simulink model "AGC30_PVcut_2021"  (R2021a)
settings: Solver=ode4  StartTime=stime  StopTime=etime  FixedStep=dtload  RelTol=1e-3
values from neighbouring files (symbols this model uses):
  AL_A = 0.3    [initset_lfc.m]
  AL_B = 0.3    [initset_lfc.m]
  DELTA_B = 0.067    [initset_otherarea.m]
  dtload = 0.1    [initset_dataload.m]
  F0 = 60    [initset_inertia.m]
  FFCS0_CC = (WF0_CC-WF_MIN_CC)./(1.0-WF_MIN_CC)    [init_thermals.m]
  FX_FB_ST_OA = Fx_fb_st_ty(:,TY_ST)    [initset_otherarea.m]
  FX_FB_WT = FX_FB_WT_ty(:,TY_WT)    [read_const_conhydros.m]
  FX_PTHD_ST_OA = Fx_pthd_st_ty(:,TY_ST)    [initset_otherarea.m]
  FY_FB_ST_OA = [1;1;0;0;-1;-1]*PLM_B    [initset_otherarea.m]
  FY_FB_WT = FY_FB_WT_ty(:,TY_WT)    [read_const_conhydros.m]
  FY_PTHD_ST_OA = [1;1;1;1]    [initset_otherarea.m]
  G_cost = [Cost(:,3) ... (first row only)    [initset_dataload.m]
  G_down_limit = max(G_down_limit, G_out_pre - G_speed*5)    [edc.m]    (also in initset_dataload.m = csvread('G_down_plan_limit.csv',0,1))
  G_G_ST_OA = G_g_st_ty(TY_ST)    [initset_otherarea.m]
  G_speed = u(220:249,1)    [edc.m]    (also in initset_dataload.m = G_speed(:,1))
  GF_CC = [1, 1, 1, 1, 1,            1, 1, 1, 1, 1]    [initset_thermals.m]
  GF_ST = [1, 1, 1, 1, 1, 1, 1,            1, 1, 1, 1,            1, 1, 1, 1, 1, 1]    [initset_thermals.m]
  GMW_WT = GMW_WT_ty(TY_WT)    [read_const_conhydros.m]
  IGV0_CC = WF0_CC    [init_thermals.m]
  inertia_input = [1 31.872 31.872 2 31.872 31.872 3 31.872 31.872 4 31.872 31.872 ... (259203 elements, 3x86401)]    [inertia_input.mat]    (also in initset_dataload.m = inertia_input')
  K1_CONV_WT = K1_CONV_WT_ty(TY_WT)    [read_const_conhydros.m]
  K2_SERV_WT = K2_SERV_WT_ty(TY_WT)    [read_const_conhydros.m]
  K_A = 0.1    [initset_lfc.m]
  K_B = 0.1    [initset_lfc.m]
  K_G_ST_OA = K_g_st_ty(TY_ST)    [initset_otherarea.m]
  K_L = 2.0    (= 2)    [initset_inertia.m]
  K_PREF_ST_OA = K_pref_st_ty(TY_ST)    [initset_otherarea.m]
  K_SD_WT = K_SD_WT_ty(TY_WT)    [read_const_conhydros.m]
  K_SEQ_WT = K_SEQ_WT_ty(TY_WT)    [read_const_conhydros.m]
  KD_PID_WT = KD_PID_WT_ty(TY_WT)    [read_const_conhydros.m]
  KGT_CC = FGT_CC./((TFR_CC-TER_CC)-(TDR_CC-TIR_CC))    [init_thermals.m]
  KI_PID_WT = KI_PID_WT_ty(TY_WT)    [read_const_conhydros.m]
  KP_A = 1.0    (= 1)    [initset_lfc.m]
  KP_B = 1.0    (= 1)    [initset_lfc.m]
  KP_PID_WT = KP_PID_WT_ty(TY_WT)    [read_const_conhydros.m]
  KST_CC = (1.0-FGT_CC)./TER_CC    [init_thermals.m]
  L_MWD_WT = L_MWD_WT_ty(TY_WT)    [read_const_conhydros.m]
  LFC_cycle = 5.0    (= 5)    [initset_lfc.m]
  load_input = load_input(:,stime+1:etime+1)    [initset_dataload.m]
  MVABase = 1000    [initset_inertia.m]
  MW0_ST = zeros(1,17)    [init_thermals.m]
  MW0_WT = zeros(1,2)    [init_conhydros.m]
  P_G_CONV_WT = P_G_CONV_WT_ty(TY_WT)    [read_const_conhydros.m]
  PG_INIT_CC = PMWD_SCHEDULE(1,19:28)'    [init_thermals.m]
  PLM_B = 0.03    [initset_otherarea.m]
  PMAX_B = 360.0    (= 360)    [initset_lfc.m]
  PMIN_B = -360.0    (= -360)    [initset_lfc.m]
  PMST0_CC = zeros(1, 10)    [init_thermals.m]
  PMWD_EDC0 = zeros(1,30)    [initset_edc.m]
  PMWD_SCHEDULE = u(3:32,1)    [edc.m]    (also in initset_edc.m = g_out_input')
  PRT_CC = PRC_CC.*(1-EP_CC)    [init_thermals.m]
  PTH0_ST = zeros(1,17)    [init_thermals.m]
  R_LL_ST_OA = R_ll_st_ty(TY_ST)    [initset_otherarea.m]
  RA_A = G_speed'    [initset_lfc.m]
  RA_B = 96.0    (= 96)    [initset_lfc.m]
  T1_B_ST_OA = T1_b_st_ty(TY_ST)    [initset_otherarea.m]
  T1_CONV_WT = T1_CONV_WT_ty(TY_WT)    [read_const_conhydros.m]
  T1_G_ST_OA = T1_g_st_ty(TY_ST)    [initset_otherarea.m]
  T2_B_ST_OA = T2_b_st_ty(TY_ST)    [initset_otherarea.m]
  T2_G_ST_OA = T2_g_st_ty(TY_ST)    [initset_otherarea.m]
  T2_SERV_WT = T2_SERV_WT_ty(TY_WT)    [read_const_conhydros.m]
  T3_B_ST_OA = T3_b_st_ty(TY_ST)    [initset_otherarea.m]
  T3_SERV_WT = T3_SERV_WT_ty(TY_WT)    [read_const_conhydros.m]
  T4_G_ST_OA = T4_g_st_ty(TY_ST)    [initset_otherarea.m]
  T5_G_ST_OA = T5_g_st_ty(TY_ST)    [initset_otherarea.m]
  T_0 = 2.5    [initset_trfpP.m]
  T_LL_ST_OA = T_ll_st_ty(TY_ST)    [initset_otherarea.m]
  T_PREF_ST_OA = T_pref_st_ty(TY_ST)    [initset_otherarea.m]
  TD_PID_WT = TD_PID_WT_ty(TY_WT)    [read_const_conhydros.m]
  TDR_CC = TIR_CC.*(1+(PRC_CC.^((RC_CC-1)./RC_CC)-1)./HC_CC)    [init_thermals.m]
  TE0_CC = zeros(1, 10)    [init_thermals.m]
  TER_CC = TFR_CC.*(1-(1-1./PRT_CC.^((RT_CC-1)./RT_CC)).*HT_CC)    [init_thermals.m]
  Tieline_Base = [1 0 2 0 3 0 4 0 5 0 6 0 ... (172802 elements, 2x86401)]    [Tieline_Base.mat]    (also in initset_dataload.m = Tieline_Base')
  TW_WAY_WT = TW_WAY_WT_ty(TY_WT)    [read_const_conhydros.m]
  U_MWD_WT = U_MWD_WT_ty(TY_WT)    [read_const_conhydros.m]
  WF0_CC = 1.0*ones(1, 10)    [init_thermals.m]
  WF_MIN_CC = L_IGV_CC./(TFR_CC-TDR_CC).*((Td_min_cc-TIR_CC)     ./((1-1./(PRT_CC.*L_IGV_CC).^((RT_CC-1)./RT_CC)).*HT_CC)-Td_min_cc)    [init_thermals.m]
  XAR_A = 10.0    (= 10)    [initset_lfc.m]
  XAR_B = 10.0    (= 10)    [initset_lfc.m]
  XF_A = 0.00    (= 0)    [initset_lfc.m]
  XF_B = 0.00    (= 0)    [initset_lfc.m]
undefined symbols (not defined in the file or in its folder): DELTA_CC, DELTA_ST, DiscIntNeverNeededParam, FGT_CC, FX_FB_CC, FX_FB_ST, FX_N_GN_VA, FX_N_PM_VA, FX_PTHD_ST, FX_T_PM_VA, FX_TE1_CC, FX_TE2_CC, FX_Y_GN_VA, FX_Y_PM_VA, FY_FB_CC, FY_FB_ST, FY_N_GN_VA, FY_N_PM_VA, FY_PTHD_ST, FY_T_PM_VA, FY_TE1_CC, FY_TE2_CC, FY_Y_GN_VA, FY_Y_PM_VA, G_G_ST, GMW_CC, GMW_ST, GMW_VA, HC_CC, HT_CC, K1_CONV_VA, K2_SERV_VA, K_G_ST, K_IGV_CC, K_MW_GV_VA, K_PREF_ST, K_SD_VA, K_TE_CC, KD_PID_VA, KD_SG_GN_VA, KD_SG_PM_VA, KI_PID_VA, KI_SG_GN_VA, KI_SG_PM_VA, KP_PID_VA, KP_SG_GN_VA, KP_SG_PM_VA, L_FUEL_CC, L_G_ST, L_IGV_CC, L_LL_ST, L_MWD_CC, L_MWD_GN_VA, L_MWD_PM_VA, L_MWD_ST, L_PREF_CC, L_PREF_ST, M_VA, MW0_ST_OA, N_GN_INIT_VA ... (+56)
libraries: simulink_extras x87, simulink x43, eeGeneralControl x2, pid_lib x1
(part 4 of 4)

== system AGC30_PVcut_2021/定速揚水発電プラント/Water1/U=1.2L=1 ==
  Inport : Inport
  Constant : Constant  Value=upper_limit
  Constant1 : Constant  Value=lower_limit
  Constant2 : Constant  Value=0
  Constant3 : Constant  Value=0
  Constant4 : Constant  Value=0
  Integrator : Integrator  InitialCondition=X0
  Logical Operator : Logic
  Logical Operator1 : Logic  Operator=OR
  Logical Operator2 : Logic  Operator=OR
  Relational operator : RelationalOperator  Operator=<=  RndMeth=Nearest  InputSameDT=on
  Relational operator1 : RelationalOperator  RndMeth=Nearest  InputSameDT=on
  Relational operator2 : RelationalOperator  Operator=<=  RndMeth=Nearest  InputSameDT=on
  Relational operator3 : RelationalOperator  RndMeth=Nearest  InputSameDT=on
  Saturation : Saturate  UpperLimit=upper_limit  LowerLimit=lower_limit
  Switch : Switch  Threshold=0.5  SaturateOnIntegerOverflow=on  InputSameDT=on
  Outport : Outport  InitialOutput=0  VectorParamsAs1DForOutWhenUnconnected=off
  wires:
  Saturation/1 -> Outport/1
  Inport/1 -> Switch/1, Relational operator2/1, Relational operator3/1
  Switch/1 -> Integrator/1
  Constant/1 -> Relational operator/2
  Constant1/1 -> Relational operator1/2
  Logical Operator/1 -> Switch/2
  Constant2/1 -> Switch/3
  Relational operator/1 -> Logical Operator1/1
  Relational operator2/1 -> Logical Operator1/2
  Logical Operator1/1 -> Logical Operator/1
  Relational operator1/1 -> Logical Operator2/1
  Relational operator3/1 -> Logical Operator2/2
  Logical Operator2/1 -> Logical Operator/2
  Constant3/1 -> Relational operator2/2
  Constant4/1 -> Relational operator3/2
  Integrator/1 -> Saturation/1, Relational operator1/1, Relational operator/1

== system AGC30_PVcut_2021/定速揚水発電プラント/Water1/U=1L=0 ==
  Inport : Inport
  Constant : Constant  Value=upper_limit
  Constant1 : Constant  Value=lower_limit
  Constant2 : Constant  Value=0
  Constant3 : Constant  Value=0
  Constant4 : Constant  Value=0
  Integrator : Integrator  InitialCondition=X0
  Logical Operator : Logic
  Logical Operator1 : Logic  Operator=OR
  Logical Operator2 : Logic  Operator=OR
  Relational operator : RelationalOperator  Operator=<=  RndMeth=Nearest  InputSameDT=on
  Relational operator1 : RelationalOperator  RndMeth=Nearest  InputSameDT=on
  Relational operator2 : RelationalOperator  Operator=<=  RndMeth=Nearest  InputSameDT=on
  Relational operator3 : RelationalOperator  RndMeth=Nearest  InputSameDT=on
  Saturation : Saturate  UpperLimit=upper_limit  LowerLimit=lower_limit
  Switch : Switch  Threshold=0.5  SaturateOnIntegerOverflow=on  InputSameDT=on
  Outport : Outport  InitialOutput=0  VectorParamsAs1DForOutWhenUnconnected=off
  wires:
  Constant4/1 -> Relational operator3/2
  Constant3/1 -> Relational operator2/2
  Logical Operator2/1 -> Logical Operator/2
  Relational operator3/1 -> Logical Operator2/2
  Relational operator1/1 -> Logical Operator2/1
  Logical Operator1/1 -> Logical Operator/1
  Relational operator2/1 -> Logical Operator1/2
  Relational operator/1 -> Logical Operator1/1
  Constant2/1 -> Switch/3
  Logical Operator/1 -> Switch/2
  Constant1/1 -> Relational operator1/2
  Constant/1 -> Relational operator/2
  Switch/1 -> Integrator/1
  Inport/1 -> Switch/1, Relational operator2/1, Relational operator3/1
  Integrator/1 -> Relational operator1/1, Relational operator/1, Saturation/1
  Saturation/1 -> Outport/1

== system AGC30_PVcut_2021/定速揚水発電プラント/Water1/連続出力切替 ==
  モデル : Inport
  運転モード : Inport  Port=2
  MWD : Inport  Port=3
  Add : Sum
  Constant : Constant  Value=0
  Gain : Gain  Gain=-1
  Gain1 : Gain  Gain=-1
  Gain2 : Gain  Gain=-1
  MWD使用時に レートを制限 : Switch  Threshold=1
  MWD使用時はMWD-モデル モデル使用時は0 : Switch  Threshold=1
  MWD使用時はMWD-モデルに追従 モデル使用時はレートでMWD-モデルから0へ変化 （MWD⇒モデル時に不連続打消し分として使用） : simulink/Discontinuities/Rate Limiter Dynamic
  Subtract : Sum  Inputs=-+
  Switch1 : Switch  Threshold=1
  ∞ : Constant  Value=9999
  モデル使用時に レートを制限 : Switch  Threshold=1
  モデル使用時はモデル-MWD MWD使用時は0 : Switch  Threshold=1
  モデル使用時はモデル-MWDに追従 MWD使用時はレートでモデル-MWDから0に変化 （モデル⇒MWD時に不連続打消し分として使用） : simulink/Discontinuities/Rate Limiter Dynamic
  不連続 打消し分 : Switch  Threshold=1
  不連続分を戻すレート : Constant  Value=0.0001
  出力 : Outport  VectorParamsAs1DForOutWhenUnconnected=off
  wires:
  MWD/1 -> Subtract/2, Switch1/3
  モデル/1 -> Switch1/1, Subtract/1
  Constant/1 -> MWD使用時はMWD-モデル モデル使用時は0/1, モデル使用時はモデル-MWD MWD使用時は0/3
  Subtract/1 -> Gain2/1, MWD使用時はMWD-モデル モデル使用時は0/3
  MWD使用時はMWD-モデル モデル使用時は0/1 -> MWD使用時はMWD-モデルに追従 モデル使用時はレートでMWD-モデルから0へ変化 （MWD⇒モデル時に不連続打消し分として使用）/2
  モデル使用時はモデル-MWD MWD使用時は0/1 -> モデル使用時はモデル-MWDに追従 MWD使用時はレートでモデル-MWDから0に変化 （モデル⇒MWD時に不連続打消し分として使用）/2
  モデル使用時はモデル-MWDに追従 MWD使用時はレートでモデル-MWDから0に変化 （モデル⇒MWD時に不連続打消し分として使用）/1 -> 不連続 打消し分/3
  MWD使用時はMWD-モデルに追従 モデル使用時はレートでMWD-モデルから0へ変化 （MWD⇒モデル時に不連続打消し分として使用）/1 -> 不連続 打消し分/1
  Add/1 -> 出力/1
  不連続分を戻すレート/1 -> モデル使用時に レートを制限/1, MWD使用時に レートを制限/3
  ∞/1 -> モデル使用時に レートを制限/3, MWD使用時に レートを制限/1
  モデル使用時に レートを制限/1 -> MWD使用時はMWD-モデルに追従 モデル使用時はレートでMWD-モデルから0へ変化 （MWD⇒モデル時に不連続打消し分として使用）/1, Gain/1
  MWD使用時に レートを制限/1 -> モデル使用時はモデル-MWDに追従 MWD使用時はレートでモデル-MWDから0に変化 （モデル⇒MWD時に不連続打消し分として使用）/1, Gain1/1
  Gain/1 -> MWD使用時はMWD-モデルに追従 モデル使用時はレートでMWD-モデルから0へ変化 （MWD⇒モデル時に不連続打消し分として使用）/3
  Gain1/1 -> モデル使用時はモデル-MWDに追従 MWD使用時はレートでモデル-MWDから0に変化 （モデル⇒MWD時に不連続打消し分として使用）/3
  Gain2/1 -> モデル使用時はモデル-MWD MWD使用時は0/1
  Switch1/1 -> Add/1
  不連続 打消し分/1 -> Add/2
  運転モード/1 -> Switch1/2, MWD使用時はMWD-モデル モデル使用時は0/2, モデル使用時はモデル-MWD MWD使用時は0/2, モデル使用時に レートを制限/2, MWD使用時に レートを制限/2, 不連続 打消し分/2

== system AGC30_PVcut_2021/定速揚水発電プラント/Water2/U=1.2L=1 ==
  Inport : Inport
  Constant : Constant  Value=upper_limit
  Constant1 : Constant  Value=lower_limit
  Constant2 : Constant  Value=0
  Constant3 : Constant  Value=0
  Constant4 : Constant  Value=0
  Integrator : Integrator  InitialCondition=X0
  Logical Operator : Logic
  Logical Operator1 : Logic  Operator=OR
  Logical Operator2 : Logic  Operator=OR
  Relational operator : RelationalOperator  Operator=<=  RndMeth=Nearest  InputSameDT=on
  Relational operator1 : RelationalOperator  RndMeth=Nearest  InputSameDT=on
  Relational operator2 : RelationalOperator  Operator=<=  RndMeth=Nearest  InputSameDT=on
  Relational operator3 : RelationalOperator  RndMeth=Nearest  InputSameDT=on
  Saturation : Saturate  UpperLimit=upper_limit  LowerLimit=lower_limit
  Switch : Switch  Threshold=0.5  SaturateOnIntegerOverflow=on  InputSameDT=on
  Outport : Outport  InitialOutput=0  VectorParamsAs1DForOutWhenUnconnected=off
  wires:
  Saturation/1 -> Outport/1
  Inport/1 -> Switch/1, Relational operator2/1, Relational operator3/1
  Switch/1 -> Integrator/1
  Constant/1 -> Relational operator/2
  Constant1/1 -> Relational operator1/2
  Logical Operator/1 -> Switch/2
  Constant2/1 -> Switch/3
  Relational operator/1 -> Logical Operator1/1
  Relational operator2/1 -> Logical Operator1/2
  Logical Operator1/1 -> Logical Operator/1
  Relational operator1/1 -> Logical Operator2/1
  Relational operator3/1 -> Logical Operator2/2
  Logical Operator2/1 -> Logical Operator/2
  Constant3/1 -> Relational operator2/2
  Constant4/1 -> Relational operator3/2
  Integrator/1 -> Saturation/1, Relational operator1/1, Relational operator/1

== system AGC30_PVcut_2021/定速揚水発電プラント/Water2/U=1L=0 ==
  Inport : Inport
  Constant : Constant  Value=upper_limit
  Constant1 : Constant  Value=lower_limit
  Constant2 : Constant  Value=0
  Constant3 : Constant  Value=0
  Constant4 : Constant  Value=0
  Integrator : Integrator  InitialCondition=X0
  Logical Operator : Logic
  Logical Operator1 : Logic  Operator=OR
  Logical Operator2 : Logic  Operator=OR
  Relational operator : RelationalOperator  Operator=<=  RndMeth=Nearest  InputSameDT=on
  Relational operator1 : RelationalOperator  RndMeth=Nearest  InputSameDT=on
  Relational operator2 : RelationalOperator  Operator=<=  RndMeth=Nearest  InputSameDT=on
  Relational operator3 : RelationalOperator  RndMeth=Nearest  InputSameDT=on
  Saturation : Saturate  UpperLimit=upper_limit  LowerLimit=lower_limit
  Switch : Switch  Threshold=0.5  SaturateOnIntegerOverflow=on  InputSameDT=on
  Outport : Outport  InitialOutput=0  VectorParamsAs1DForOutWhenUnconnected=off
  wires:
  Constant4/1 -> Relational operator3/2
  Constant3/1 -> Relational operator2/2
  Logical Operator2/1 -> Logical Operator/2
  Relational operator3/1 -> Logical Operator2/2
  Relational operator1/1 -> Logical Operator2/1
  Logical Operator1/1 -> Logical Operator/1
  Relational operator2/1 -> Logical Operator1/2
  Relational operator/1 -> Logical Operator1/1
  Constant2/1 -> Switch/3
  Logical Operator/1 -> Switch/2
  Constant1/1 -> Relational operator1/2
  Constant/1 -> Relational operator/2
  Switch/1 -> Integrator/1
  Inport/1 -> Switch/1, Relational operator2/1, Relational operator3/1
  Integrator/1 -> Relational operator1/1, Relational operator/1, Saturation/1
  Saturation/1 -> Outport/1

== system AGC30_PVcut_2021/定速揚水発電プラント/Water2/連続出力切替 ==
  モデル : Inport
  運転モード : Inport  Port=2
  MWD : Inport  Port=3
  Add : Sum
  Constant : Constant  Value=0
  Gain : Gain  Gain=-1
  Gain1 : Gain  Gain=-1
  Gain2 : Gain  Gain=-1
  MWD使用時に レートを制限 : Switch  Threshold=1
  MWD使用時はMWD-モデル モデル使用時は0 : Switch  Threshold=1
  MWD使用時はMWD-モデルに追従 モデル使用時はレートでMWD-モデルから0へ変化 （MWD⇒モデル時に不連続打消し分として使用） : simulink/Discontinuities/Rate Limiter Dynamic
  Subtract : Sum  Inputs=-+
  Switch1 : Switch  Threshold=1
  ∞ : Constant  Value=9999
  モデル使用時に レートを制限 : Switch  Threshold=1
  モデル使用時はモデル-MWD MWD使用時は0 : Switch  Threshold=1
  モデル使用時はモデル-MWDに追従 MWD使用時はレートでモデル-MWDから0に変化 （モデル⇒MWD時に不連続打消し分として使用） : simulink/Discontinuities/Rate Limiter Dynamic
  不連続 打消し分 : Switch  Threshold=1
  不連続分を戻すレート : Constant  Value=0.0001
  出力 : Outport  VectorParamsAs1DForOutWhenUnconnected=off
  wires:
  MWD/1 -> Subtract/2, Switch1/3
  モデル/1 -> Switch1/1, Subtract/1
  Constant/1 -> MWD使用時はMWD-モデル モデル使用時は0/1, モデル使用時はモデル-MWD MWD使用時は0/3
  Subtract/1 -> Gain2/1, MWD使用時はMWD-モデル モデル使用時は0/3
  MWD使用時はMWD-モデル モデル使用時は0/1 -> MWD使用時はMWD-モデルに追従 モデル使用時はレートでMWD-モデルから0へ変化 （MWD⇒モデル時に不連続打消し分として使用）/2
  モデル使用時はモデル-MWD MWD使用時は0/1 -> モデル使用時はモデル-MWDに追従 MWD使用時はレートでモデル-MWDから0に変化 （モデル⇒MWD時に不連続打消し分として使用）/2
  モデル使用時はモデル-MWDに追従 MWD使用時はレートでモデル-MWDから0に変化 （モデル⇒MWD時に不連続打消し分として使用）/1 -> 不連続 打消し分/3
  MWD使用時はMWD-モデルに追従 モデル使用時はレートでMWD-モデルから0へ変化 （MWD⇒モデル時に不連続打消し分として使用）/1 -> 不連続 打消し分/1
  Add/1 -> 出力/1
  不連続分を戻すレート/1 -> モデル使用時に レートを制限/1, MWD使用時に レートを制限/3
  ∞/1 -> モデル使用時に レートを制限/3, MWD使用時に レートを制限/1
  モデル使用時に レートを制限/1 -> MWD使用時はMWD-モデルに追従 モデル使用時はレートでMWD-モデルから0へ変化 （MWD⇒モデル時に不連続打消し分として使用）/1, Gain/1
  MWD使用時に レートを制限/1 -> モデル使用時はモデル-MWDに追従 MWD使用時はレートでモデル-MWDから0に変化 （モデル⇒MWD時に不連続打消し分として使用）/1, Gain1/1
  Gain/1 -> MWD使用時はMWD-モデルに追従 モデル使用時はレートでMWD-モデルから0へ変化 （MWD⇒モデル時に不連続打消し分として使用）/3
  Gain1/1 -> モデル使用時はモデル-MWDに追従 MWD使用時はレートでモデル-MWDから0に変化 （モデル⇒MWD時に不連続打消し分として使用）/3
  Gain2/1 -> モデル使用時はモデル-MWD MWD使用時は0/1
  Switch1/1 -> Add/1
  不連続 打消し分/1 -> Add/2
  運転モード/1 -> Switch1/2, MWD使用時はMWD-モデル モデル使用時は0/2, モデル使用時はモデル-MWD MWD使用時は0/2, モデル使用時に レートを制限/2, MWD使用時に レートを制限/2, 不連続 打消し分/2

== system AGC30_PVcut_2021/汽力プラント/Coal1/追従回路 ==
  In : Inport
  Subtract2 : Sum  Inputs=+-
  追従回路積分1 : Integrator  InitialCondition=MW0_ST(8)/PTH0_ST(8)+PLM_ST(8)  LimitOutput=on  UpperSaturationLimit=U_LL_ST(8)  LowerSaturationLimit=L_LL_ST(8)
  追従変化率 : Saturate  UpperLimit=R_LL_ST(8)/60  LowerLimit=-R_LL_ST(8)/60
  追従時定数 : Gain  Gain=1/T_LL_ST(8)
  Out : Outport  VectorParamsAs1DForOutWhenUnconnected=off
  wires:
  Subtract2/1 -> 追従時定数/1
  追従時定数/1 -> 追従変化率/1
  追従変化率/1 -> 追従回路積分1/1
  追従回路積分1/1 -> Out/1, Subtract2/2
  In/1 -> Subtract2/1

== system AGC30_PVcut_2021/汽力プラント/Coal1/連続出力切替 ==
  モデル : Inport
  運転モード : Inport  Port=2
  MWD : Inport  Port=3
  Add : Sum
  Constant : Constant  Value=0
  Gain : Gain  Gain=-1
  Gain1 : Gain  Gain=-1
  Gain2 : Gain  Gain=-1
  MWD使用時に レートを制限 : Switch  Threshold=1
  MWD使用時はMWD-モデル モデル使用時は0 : Switch  Threshold=1
  MWD使用時はMWD-モデルに追従 モデル使用時はレートでMWD-モデルから0へ変化 （MWD⇒モデル時に不連続打消し分として使用） : simulink/Discontinuities/Rate Limiter Dynamic
  Subtract : Sum  Inputs=-+
  Switch1 : Switch  Threshold=1
  ∞ : Constant  Value=9999
  モデル使用時に レートを制限 : Switch  Threshold=1
  モデル使用時はモデル-MWD MWD使用時は0 : Switch  Threshold=1
  モデル使用時はモデル-MWDに追従 MWD使用時はレートでモデル-MWDから0に変化 （モデル⇒MWD時に不連続打消し分として使用） : simulink/Discontinuities/Rate Limiter Dynamic
  不連続 打消し分 : Switch  Threshold=1
  不連続分を戻すレート : Constant  Value=0.0001
  出力 : Outport  VectorParamsAs1DForOutWhenUnconnected=off
  wires:
  MWD/1 -> Subtract/2, Switch1/3
  モデル/1 -> Switch1/1, Subtract/1
  Constant/1 -> MWD使用時はMWD-モデル モデル使用時は0/1, モデル使用時はモデル-MWD MWD使用時は0/3
  Subtract/1 -> Gain2/1, MWD使用時はMWD-モデル モデル使用時は0/3
  MWD使用時はMWD-モデル モデル使用時は0/1 -> MWD使用時はMWD-モデルに追従 モデル使用時はレートでMWD-モデルから0へ変化 （MWD⇒モデル時に不連続打消し分として使用）/2
  モデル使用時はモデル-MWD MWD使用時は0/1 -> モデル使用時はモデル-MWDに追従 MWD使用時はレートでモデル-MWDから0に変化 （モデル⇒MWD時に不連続打消し分として使用）/2
  モデル使用時はモデル-MWDに追従 MWD使用時はレートでモデル-MWDから0に変化 （モデル⇒MWD時に不連続打消し分として使用）/1 -> 不連続 打消し分/3
  MWD使用時はMWD-モデルに追従 モデル使用時はレートでMWD-モデルから0へ変化 （MWD⇒モデル時に不連続打消し分として使用）/1 -> 不連続 打消し分/1
  Add/1 -> 出力/1
  不連続分を戻すレート/1 -> モデル使用時に レートを制限/1, MWD使用時に レートを制限/3
  ∞/1 -> モデル使用時に レートを制限/3, MWD使用時に レートを制限/1
  モデル使用時に レートを制限/1 -> MWD使用時はMWD-モデルに追従 モデル使用時はレートでMWD-モデルから0へ変化 （MWD⇒モデル時に不連続打消し分として使用）/1, Gain/1
  MWD使用時に レートを制限/1 -> モデル使用時はモデル-MWDに追従 MWD使用時はレートでモデル-MWDから0に変化 （モデル⇒MWD時に不連続打消し分として使用）/1, Gain1/1
  Gain/1 -> MWD使用時はMWD-モデルに追従 モデル使用時はレートでMWD-モデルから0へ変化 （MWD⇒モデル時に不連続打消し分として使用）/3
  Gain1/1 -> モデル使用時はモデル-MWDに追従 MWD使用時はレートでモデル-MWDから0に変化 （モデル⇒MWD時に不連続打消し分として使用）/3
  Gain2/1 -> モデル使用時はモデル-MWD MWD使用時は0/1
  Switch1/1 -> Add/1
  不連続 打消し分/1 -> Add/2
  運転モード/1 -> Switch1/2, MWD使用時はMWD-モデル モデル使用時は0/2, モデル使用時はモデル-MWD MWD使用時は0/2, モデル使用時に レートを制限/2, MWD使用時に レートを制限/2, 不連続 打消し分/2

== system AGC30_PVcut_2021/汽力プラント/Coal2/追従回路 ==
  In : Inport
  Subtract2 : Sum  Inputs=+-
  追従回路積分1 : Integrator  InitialCondition=MW0_ST(8)/PTH0_ST(8)+PLM_ST(8)  LimitOutput=on  UpperSaturationLimit=U_LL_ST(8)  LowerSaturationLimit=L_LL_ST(8)
  追従変化率 : Saturate  UpperLimit=R_LL_ST(8)/60  LowerLimit=-R_LL_ST(8)/60
  追従時定数 : Gain  Gain=1/T_LL_ST(8)
  Out : Outport  VectorParamsAs1DForOutWhenUnconnected=off
  wires:
  In/1 -> Subtract2/1
  追従回路積分1/1 -> Subtract2/2, Out/1
  追従変化率/1 -> 追従回路積分1/1
  追従時定数/1 -> 追従変化率/1
  Subtract2/1 -> 追従時定数/1

== system AGC30_PVcut_2021/汽力プラント/Coal2/連続出力切替 ==
  モデル : Inport
  運転モード : Inport  Port=2
  MWD : Inport  Port=3
  Add : Sum
  Constant : Constant  Value=0
  Gain : Gain  Gain=-1
  Gain1 : Gain  Gain=-1
  Gain2 : Gain  Gain=-1
  MWD使用時に レートを制限 : Switch  Threshold=1
  MWD使用時はMWD-モデル モデル使用時は0 : Switch  Threshold=1
  MWD使用時はMWD-モデルに追従 モデル使用時はレートでMWD-モデルから0へ変化 （MWD⇒モデル時に不連続打消し分として使用） : simulink/Discontinuities/Rate Limiter Dynamic
  Subtract : Sum  Inputs=-+
  Switch1 : Switch  Threshold=1
  ∞ : Constant  Value=9999
  モデル使用時に レートを制限 : Switch  Threshold=1
  モデル使用時はモデル-MWD MWD使用時は0 : Switch  Threshold=1
  モデル使用時はモデル-MWDに追従 MWD使用時はレートでモデル-MWDから0に変化 （モデル⇒MWD時に不連続打消し分として使用） : simulink/Discontinuities/Rate Limiter Dynamic
  不連続 打消し分 : Switch  Threshold=1
  不連続分を戻すレート : Constant  Value=0.0001
  出力 : Outport  VectorParamsAs1DForOutWhenUnconnected=off
  wires:
  運転モード/1 -> 不連続 打消し分/2, MWD使用時に レートを制限/2, モデル使用時に レートを制限/2, モデル使用時はモデル-MWD MWD使用時は0/2, MWD使用時はMWD-モデル モデル使用時は0/2, Switch1/2
  不連続 打消し分/1 -> Add/2
  Switch1/1 -> Add/1
  Gain2/1 -> モデル使用時はモデル-MWD MWD使用時は0/1
  Gain1/1 -> モデル使用時はモデル-MWDに追従 MWD使用時はレートでモデル-MWDから0に変化 （モデル⇒MWD時に不連続打消し分として使用）/3
  Gain/1 -> MWD使用時はMWD-モデルに追従 モデル使用時はレートでMWD-モデルから0へ変化 （MWD⇒モデル時に不連続打消し分として使用）/3
  MWD使用時に レートを制限/1 -> Gain1/1, モデル使用時はモデル-MWDに追従 MWD使用時はレートでモデル-MWDから0に変化 （モデル⇒MWD時に不連続打消し分として使用）/1
  モデル使用時に レートを制限/1 -> Gain/1, MWD使用時はMWD-モデルに追従 モデル使用時はレートでMWD-モデルから0へ変化 （MWD⇒モデル時に不連続打消し分として使用）/1
  ∞/1 -> MWD使用時に レートを制限/1, モデル使用時に レートを制限/3
  不連続分を戻すレート/1 -> MWD使用時に レートを制限/3, モデル使用時に レートを制限/1
  Add/1 -> 出力/1
  MWD使用時はMWD-モデルに追従 モデル使用時はレートでMWD-モデルから0へ変化 （MWD⇒モデル時に不連続打消し分として使用）/1 -> 不連続 打消し分/1
  モデル使用時はモデル-MWDに追従 MWD使用時はレートでモデル-MWDから0に変化 （モデル⇒MWD時に不連続打消し分として使用）/1 -> 不連続 打消し分/3
  モデル使用時はモデル-MWD MWD使用時は0/1 -> モデル使用時はモデル-MWDに追従 MWD使用時はレートでモデル-MWDから0に変化 （モデル⇒MWD時に不連続打消し分として使用）/2
  MWD使用時はMWD-モデル モデル使用時は0/1 -> MWD使用時はMWD-モデルに追従 モデル使用時はレートでMWD-モデルから0へ変化 （MWD⇒モデル時に不連続打消し分として使用）/2
  Subtract/1 -> MWD使用時はMWD-モデル モデル使用時は0/3, Gain2/1
  Constant/1 -> モデル使用時はモデル-MWD MWD使用時は0/3, MWD使用時はMWD-モデル モデル使用時は0/1
  モデル/1 -> Subtract/1, Switch1/1
  MWD/1 -> Switch1/3, Subtract/2

== system AGC30_PVcut_2021/汽力プラント/Coal3/追従回路 ==
  In : Inport
  Subtract2 : Sum  Inputs=+-
  追従回路積分1 : Integrator  InitialCondition=MW0_ST(8)/PTH0_ST(8)+PLM_ST(8)  LimitOutput=on  UpperSaturationLimit=U_LL_ST(8)  LowerSaturationLimit=L_LL_ST(8)
  追従変化率 : Saturate  UpperLimit=R_LL_ST(8)/60  LowerLimit=-R_LL_ST(8)/60
  追従時定数 : Gain  Gain=1/T_LL_ST(8)
  Out : Outport  VectorParamsAs1DForOutWhenUnconnected=off
  wires:
  Subtract2/1 -> 追従時定数/1
  追従時定数/1 -> 追従変化率/1
  追従変化率/1 -> 追従回路積分1/1
  追従回路積分1/1 -> Out/1, Subtract2/2
  In/1 -> Subtract2/1

== system AGC30_PVcut_2021/汽力プラント/Coal3/連続出力切替 ==
  モデル : Inport
  運転モード : Inport  Port=2
  MWD : Inport  Port=3
  Add : Sum
  Constant : Constant  Value=0
  Gain : Gain  Gain=-1
  Gain1 : Gain  Gain=-1
  Gain2 : Gain  Gain=-1
  MWD使用時に レートを制限 : Switch  Threshold=1
  MWD使用時はMWD-モデル モデル使用時は0 : Switch  Threshold=1
  MWD使用時はMWD-モデルに追従 モデル使用時はレートでMWD-モデルから0へ変化 （MWD⇒モデル時に不連続打消し分として使用） : simulink/Discontinuities/Rate Limiter Dynamic
  Subtract : Sum  Inputs=-+
  Switch1 : Switch  Threshold=1
  ∞ : Constant  Value=9999
  モデル使用時に レートを制限 : Switch  Threshold=1
  モデル使用時はモデル-MWD MWD使用時は0 : Switch  Threshold=1
  モデル使用時はモデル-MWDに追従 MWD使用時はレートでモデル-MWDから0に変化 （モデル⇒MWD時に不連続打消し分として使用） : simulink/Discontinuities/Rate Limiter Dynamic
  不連続 打消し分 : Switch  Threshold=1
  不連続分を戻すレート : Constant  Value=0.0001
  出力 : Outport  VectorParamsAs1DForOutWhenUnconnected=off
  wires:
  MWD/1 -> Subtract/2, Switch1/3
  モデル/1 -> Switch1/1, Subtract/1
  Constant/1 -> MWD使用時はMWD-モデル モデル使用時は0/1, モデル使用時はモデル-MWD MWD使用時は0/3
  Subtract/1 -> Gain2/1, MWD使用時はMWD-モデル モデル使用時は0/3
  MWD使用時はMWD-モデル モデル使用時は0/1 -> MWD使用時はMWD-モデルに追従 モデル使用時はレートでMWD-モデルから0へ変化 （MWD⇒モデル時に不連続打消し分として使用）/2
  モデル使用時はモデル-MWD MWD使用時は0/1 -> モデル使用時はモデル-MWDに追従 MWD使用時はレートでモデル-MWDから0に変化 （モデル⇒MWD時に不連続打消し分として使用）/2
  モデル使用時はモデル-MWDに追従 MWD使用時はレートでモデル-MWDから0に変化 （モデル⇒MWD時に不連続打消し分として使用）/1 -> 不連続 打消し分/3
  MWD使用時はMWD-モデルに追従 モデル使用時はレートでMWD-モデルから0へ変化 （MWD⇒モデル時に不連続打消し分として使用）/1 -> 不連続 打消し分/1
  Add/1 -> 出力/1
  不連続分を戻すレート/1 -> モデル使用時に レートを制限/1, MWD使用時に レートを制限/3
  ∞/1 -> モデル使用時に レートを制限/3, MWD使用時に レートを制限/1
  モデル使用時に レートを制限/1 -> MWD使用時はMWD-モデルに追従 モデル使用時はレートでMWD-モデルから0へ変化 （MWD⇒モデル時に不連続打消し分として使用）/1, Gain/1
  MWD使用時に レートを制限/1 -> モデル使用時はモデル-MWDに追従 MWD使用時はレートでモデル-MWDから0に変化 （モデル⇒MWD時に不連続打消し分として使用）/1, Gain1/1
  Gain/1 -> MWD使用時はMWD-モデルに追従 モデル使用時はレートでMWD-モデルから0へ変化 （MWD⇒モデル時に不連続打消し分として使用）/3
  Gain1/1 -> モデル使用時はモデル-MWDに追従 MWD使用時はレートでモデル-MWDから0に変化 （モデル⇒MWD時に不連続打消し分として使用）/3
  Gain2/1 -> モデル使用時はモデル-MWD MWD使用時は0/1
  Switch1/1 -> Add/1
  不連続 打消し分/1 -> Add/2
  運転モード/1 -> Switch1/2, MWD使用時はMWD-モデル モデル使用時は0/2, モデル使用時はモデル-MWD MWD使用時は0/2, モデル使用時に レートを制限/2, MWD使用時に レートを制限/2, 不連続 打消し分/2

== system AGC30_PVcut_2021/汽力プラント/Coal4/追従回路 ==
  In : Inport
  Subtract2 : Sum  Inputs=+-
  追従回路積分1 : Integrator  InitialCondition=MW0_ST(9)/PTH0_ST(9)+PLM_ST(9)  LimitOutput=on  UpperSaturationLimit=U_LL_ST(9)  LowerSaturationLimit=L_LL_ST(9)
  追従変化率 : Saturate  UpperLimit=R_LL_ST(9)/60  LowerLimit=-R_LL_ST(9)/60
  追従時定数 : Gain  Gain=1/T_LL_ST(9)
  Out : Outport  VectorParamsAs1DForOutWhenUnconnected=off
  wires:
  Subtract2/1 -> 追従時定数/1
  追従時定数/1 -> 追従変化率/1
  追従変化率/1 -> 追従回路積分1/1
  追従回路積分1/1 -> Out/1, Subtract2/2
  In/1 -> Subtract2/1

== system AGC30_PVcut_2021/汽力プラント/Coal4/連続出力切替 ==
  モデル : Inport
  運転モード : Inport  Port=2
  MWD : Inport  Port=3
  Add : Sum
  Constant : Constant  Value=0
  Gain : Gain  Gain=-1
  Gain1 : Gain  Gain=-1
  Gain2 : Gain  Gain=-1
  MWD使用時に レートを制限 : Switch  Threshold=1
  MWD使用時はMWD-モデル モデル使用時は0 : Switch  Threshold=1
  MWD使用時はMWD-モデルに追従 モデル使用時はレートでMWD-モデルから0へ変化 （MWD⇒モデル時に不連続打消し分として使用） : simulink/Discontinuities/Rate Limiter Dynamic
  Subtract : Sum  Inputs=-+
  Switch1 : Switch  Threshold=1
  ∞ : Constant  Value=9999
  モデル使用時に レートを制限 : Switch  Threshold=1
  モデル使用時はモデル-MWD MWD使用時は0 : Switch  Threshold=1
  モデル使用時はモデル-MWDに追従 MWD使用時はレートでモデル-MWDから0に変化 （モデル⇒MWD時に不連続打消し分として使用） : simulink/Discontinuities/Rate Limiter Dynamic
  不連続 打消し分 : Switch  Threshold=1
  不連続分を戻すレート : Constant  Value=0.0001
  出力 : Outport  VectorParamsAs1DForOutWhenUnconnected=off
  wires:
  MWD/1 -> Subtract/2, Switch1/3
  モデル/1 -> Switch1/1, Subtract/1
  Constant/1 -> MWD使用時はMWD-モデル モデル使用時は0/1, モデル使用時はモデル-MWD MWD使用時は0/3
  Subtract/1 -> Gain2/1, MWD使用時はMWD-モデル モデル使用時は0/3
  MWD使用時はMWD-モデル モデル使用時は0/1 -> MWD使用時はMWD-モデルに追従 モデル使用時はレートでMWD-モデルから0へ変化 （MWD⇒モデル時に不連続打消し分として使用）/2
  モデル使用時はモデル-MWD MWD使用時は0/1 -> モデル使用時はモデル-MWDに追従 MWD使用時はレートでモデル-MWDから0に変化 （モデル⇒MWD時に不連続打消し分として使用）/2
  モデル使用時はモデル-MWDに追従 MWD使用時はレートでモデル-MWDから0に変化 （モデル⇒MWD時に不連続打消し分として使用）/1 -> 不連続 打消し分/3
  MWD使用時はMWD-モデルに追従 モデル使用時はレートでMWD-モデルから0へ変化 （MWD⇒モデル時に不連続打消し分として使用）/1 -> 不連続 打消し分/1
  Add/1 -> 出力/1
  不連続分を戻すレート/1 -> モデル使用時に レートを制限/1, MWD使用時に レートを制限/3
  ∞/1 -> モデル使用時に レートを制限/3, MWD使用時に レートを制限/1
  モデル使用時に レートを制限/1 -> MWD使用時はMWD-モデルに追従 モデル使用時はレートでMWD-モデルから0へ変化 （MWD⇒モデル時に不連続打消し分として使用）/1, Gain/1
  MWD使用時に レートを制限/1 -> モデル使用時はモデル-MWDに追従 MWD使用時はレートでモデル-MWDから0に変化 （モデル⇒MWD時に不連続打消し分として使用）/1, Gain1/1
  Gain/1 -> MWD使用時はMWD-モデルに追従 モデル使用時はレートでMWD-モデルから0へ変化 （MWD⇒モデル時に不連続打消し分として使用）/3
  Gain1/1 -> モデル使用時はモデル-MWDに追従 MWD使用時はレートでモデル-MWDから0に変化 （モデル⇒MWD時に不連続打消し分として使用）/3
  Gain2/1 -> モデル使用時はモデル-MWD MWD使用時は0/1
  Switch1/1 -> Add/1
  不連続 打消し分/1 -> Add/2
  運転モード/1 -> Switch1/2, MWD使用時はMWD-モデル モデル使用時は0/2, モデル使用時はモデル-MWD MWD使用時は0/2, モデル使用時に レートを制限/2, MWD使用時に レートを制限/2, 不連続 打消し分/2

== system AGC30_PVcut_2021/汽力プラント/Coal5/追従回路 ==
  In : Inport
  Subtract2 : Sum  Inputs=+-
  追従回路積分1 : Integrator  InitialCondition=MW0_ST(10)/PTH0_ST(10)+PLM_ST(10)  LimitOutput=on  UpperSaturationLimit=U_LL_ST(10)  LowerSaturationLimit=L_LL_ST(10)
  追従変化率 : Saturate  UpperLimit=R_LL_ST(10)/60  LowerLimit=-R_LL_ST(10)/60
  追従時定数 : Gain  Gain=1/T_LL_ST(10)
  Out : Outport  VectorParamsAs1DForOutWhenUnconnected=off
  wires:
  Subtract2/1 -> 追従時定数/1
  追従時定数/1 -> 追従変化率/1
  追従変化率/1 -> 追従回路積分1/1
  追従回路積分1/1 -> Out/1, Subtract2/2
  In/1 -> Subtract2/1

== system AGC30_PVcut_2021/汽力プラント/Coal5/連続出力切替 ==
  モデル : Inport
  運転モード : Inport  Port=2
  MWD : Inport  Port=3
  Add : Sum
  Constant : Constant  Value=0
  Gain : Gain  Gain=-1
  Gain1 : Gain  Gain=-1
  Gain2 : Gain  Gain=-1
  MWD使用時に レートを制限 : Switch  Threshold=1
  MWD使用時はMWD-モデル モデル使用時は0 : Switch  Threshold=1
  MWD使用時はMWD-モデルに追従 モデル使用時はレートでMWD-モデルから0へ変化 （MWD⇒モデル時に不連続打消し分として使用） : simulink/Discontinuities/Rate Limiter Dynamic
  Subtract : Sum  Inputs=-+
  Switch1 : Switch  Threshold=1
  ∞ : Constant  Value=9999
  モデル使用時に レートを制限 : Switch  Threshold=1
  モデル使用時はモデル-MWD MWD使用時は0 : Switch  Threshold=1
  モデル使用時はモデル-MWDに追従 MWD使用時はレートでモデル-MWDから0に変化 （モデル⇒MWD時に不連続打消し分として使用） : simulink/Discontinuities/Rate Limiter Dynamic
  不連続 打消し分 : Switch  Threshold=1
  不連続分を戻すレート : Constant  Value=0.0001
  出力 : Outport  VectorParamsAs1DForOutWhenUnconnected=off
  wires:
  MWD/1 -> Subtract/2, Switch1/3
  モデル/1 -> Switch1/1, Subtract/1
  Constant/1 -> MWD使用時はMWD-モデル モデル使用時は0/1, モデル使用時はモデル-MWD MWD使用時は0/3
  Subtract/1 -> Gain2/1, MWD使用時はMWD-モデル モデル使用時は0/3
  MWD使用時はMWD-モデル モデル使用時は0/1 -> MWD使用時はMWD-モデルに追従 モデル使用時はレートでMWD-モデルから0へ変化 （MWD⇒モデル時に不連続打消し分として使用）/2
  モデル使用時はモデル-MWD MWD使用時は0/1 -> モデル使用時はモデル-MWDに追従 MWD使用時はレートでモデル-MWDから0に変化 （モデル⇒MWD時に不連続打消し分として使用）/2
  モデル使用時はモデル-MWDに追従 MWD使用時はレートでモデル-MWDから0に変化 （モデル⇒MWD時に不連続打消し分として使用）/1 -> 不連続 打消し分/3
  MWD使用時はMWD-モデルに追従 モデル使用時はレートでMWD-モデルから0へ変化 （MWD⇒モデル時に不連続打消し分として使用）/1 -> 不連続 打消し分/1
  Add/1 -> 出力/1
  不連続分を戻すレート/1 -> モデル使用時に レートを制限/1, MWD使用時に レートを制限/3
  ∞/1 -> モデル使用時に レートを制限/3, MWD使用時に レートを制限/1
  モデル使用時に レートを制限/1 -> MWD使用時はMWD-モデルに追従 モデル使用時はレートでMWD-モデルから0へ変化 （MWD⇒モデル時に不連続打消し分として使用）/1, Gain/1
  MWD使用時に レートを制限/1 -> モデル使用時はモデル-MWDに追従 MWD使用時はレートでモデル-MWDから0に変化 （モデル⇒MWD時に不連続打消し分として使用）/1, Gain1/1
  Gain/1 -> MWD使用時はMWD-モデルに追従 モデル使用時はレートでMWD-モデルから0へ変化 （MWD⇒モデル時に不連続打消し分として使用）/3
  Gain1/1 -> モデル使用時はモデル-MWDに追従 MWD使用時はレートでモデル-MWDから0に変化 （モデル⇒MWD時に不連続打消し分として使用）/3
  Gain2/1 -> モデル使用時はモデル-MWD MWD使用時は0/1
  Switch1/1 -> Add/1
  不連続 打消し分/1 -> Add/2
  運転モード/1 -> Switch1/2, MWD使用時はMWD-モデル モデル使用時は0/2, モデル使用時はモデル-MWD MWD使用時は0/2, モデル使用時に レートを制限/2, MWD使用時に レートを制限/2, 不連続 打消し分/2

== system AGC30_PVcut_2021/汽力プラント/Coal6/追従回路 ==
  In : Inport
  Subtract2 : Sum  Inputs=+-
  追従回路積分1 : Integrator  InitialCondition=MW0_ST(11)/PTH0_ST(11)+PLM_ST(11)  LimitOutput=on  UpperSaturationLimit=U_LL_ST(11)  LowerSaturationLimit=L_LL_ST(11)
  追従変化率 : Saturate  UpperLimit=R_LL_ST(11)/60  LowerLimit=-R_LL_ST(11)/60
  追従時定数 : Gain  Gain=1/T_LL_ST(11)
  Out : Outport  VectorParamsAs1DForOutWhenUnconnected=off
  wires:
  Subtract2/1 -> 追従時定数/1
  追従時定数/1 -> 追従変化率/1
  追従変化率/1 -> 追従回路積分1/1
  追従回路積分1/1 -> Out/1, Subtract2/2
  In/1 -> Subtract2/1

== system AGC30_PVcut_2021/汽力プラント/Coal6/連続出力切替 ==
  モデル : Inport
  運転モード : Inport  Port=2
  MWD : Inport  Port=3
  Add : Sum
  Constant : Constant  Value=0
  Gain : Gain  Gain=-1
  Gain1 : Gain  Gain=-1
  Gain2 : Gain  Gain=-1
  MWD使用時に レートを制限 : Switch  Threshold=1
  MWD使用時はMWD-モデル モデル使用時は0 : Switch  Threshold=1
  MWD使用時はMWD-モデルに追従 モデル使用時はレートでMWD-モデルから0へ変化 （MWD⇒モデル時に不連続打消し分として使用） : simulink/Discontinuities/Rate Limiter Dynamic
  Subtract : Sum  Inputs=-+
  Switch1 : Switch  Threshold=1
  ∞ : Constant  Value=9999
  モデル使用時に レートを制限 : Switch  Threshold=1
  モデル使用時はモデル-MWD MWD使用時は0 : Switch  Threshold=1
  モデル使用時はモデル-MWDに追従 MWD使用時はレートでモデル-MWDから0に変化 （モデル⇒MWD時に不連続打消し分として使用） : simulink/Discontinuities/Rate Limiter Dynamic
  不連続 打消し分 : Switch  Threshold=1
  不連続分を戻すレート : Constant  Value=0.0001
  出力 : Outport  VectorParamsAs1DForOutWhenUnconnected=off
  wires:
  MWD/1 -> Subtract/2, Switch1/3
  モデル/1 -> Switch1/1, Subtract/1
  Constant/1 -> MWD使用時はMWD-モデル モデル使用時は0/1, モデル使用時はモデル-MWD MWD使用時は0/3
  Subtract/1 -> Gain2/1, MWD使用時はMWD-モデル モデル使用時は0/3
  MWD使用時はMWD-モデル モデル使用時は0/1 -> MWD使用時はMWD-モデルに追従 モデル使用時はレートでMWD-モデルから0へ変化 （MWD⇒モデル時に不連続打消し分として使用）/2
  モデル使用時はモデル-MWD MWD使用時は0/1 -> モデル使用時はモデル-MWDに追従 MWD使用時はレートでモデル-MWDから0に変化 （モデル⇒MWD時に不連続打消し分として使用）/2
  モデル使用時はモデル-MWDに追従 MWD使用時はレートでモデル-MWDから0に変化 （モデル⇒MWD時に不連続打消し分として使用）/1 -> 不連続 打消し分/3
  MWD使用時はMWD-モデルに追従 モデル使用時はレートでMWD-モデルから0へ変化 （MWD⇒モデル時に不連続打消し分として使用）/1 -> 不連続 打消し分/1
  Add/1 -> 出力/1
  不連続分を戻すレート/1 -> モデル使用時に レートを制限/1, MWD使用時に レートを制限/3
  ∞/1 -> モデル使用時に レートを制限/3, MWD使用時に レートを制限/1
  モデル使用時に レートを制限/1 -> MWD使用時はMWD-モデルに追従 モデル使用時はレートでMWD-モデルから0へ変化 （MWD⇒モデル時に不連続打消し分として使用）/1, Gain/1
  MWD使用時に レートを制限/1 -> モデル使用時はモデル-MWDに追従 MWD使用時はレートでモデル-MWDから0に変化 （モデル⇒MWD時に不連続打消し分として使用）/1, Gain1/1
  Gain/1 -> MWD使用時はMWD-モデルに追従 モデル使用時はレートでMWD-モデルから0へ変化 （MWD⇒モデル時に不連続打消し分として使用）/3
  Gain1/1 -> モデル使用時はモデル-MWDに追従 MWD使用時はレートでモデル-MWDから0に変化 （モデル⇒MWD時に不連続打消し分として使用）/3
  Gain2/1 -> モデル使用時はモデル-MWD MWD使用時は0/1
  Switch1/1 -> Add/1
  不連続 打消し分/1 -> Add/2
  運転モード/1 -> Switch1/2, MWD使用時はMWD-モデル モデル使用時は0/2, モデル使用時はモデル-MWD MWD使用時は0/2, モデル使用時に レートを制限/2, MWD使用時に レートを制限/2, 不連続 打消し分/2

== system AGC30_PVcut_2021/汽力プラント/Oil1/追従回路 ==
  In : Inport
  Subtract2 : Sum  Inputs=+-
  追従回路積分 : Integrator  InitialCondition=MW0_ST(1)/PTH0_ST(1)+PLM_ST(1)  LimitOutput=on  UpperSaturationLimit=U_LL_ST(1)  LowerSaturationLimit=L_LL_ST(1)
  追従変化率 : Saturate  UpperLimit=R_LL_ST(1)/60  LowerLimit=-R_LL_ST(1)/60
  追従時定数 : Gain  Gain=1/T_LL_ST(1)
  Out : Outport  VectorParamsAs1DForOutWhenUnconnected=off
  wires:
  Subtract2/1 -> 追従時定数/1
  追従時定数/1 -> 追従変化率/1
  追従変化率/1 -> 追従回路積分/1
  追従回路積分/1 -> Out/1, Subtract2/2
  In/1 -> Subtract2/1

== system AGC30_PVcut_2021/汽力プラント/Oil1/連続出力切替 ==
  モデル : Inport
  運転モード : Inport  Port=2
  MWD : Inport  Port=3
  Add : Sum
  Constant : Constant  Value=0
  Gain : Gain  Gain=-1
  Gain1 : Gain  Gain=-1
  Gain2 : Gain  Gain=-1
  MWD使用時に レートを制限 : Switch  Threshold=1
  MWD使用時はMWD-モデル モデル使用時は0 : Switch  Threshold=1
  MWD使用時はMWD-モデルに追従 モデル使用時はレートでMWD-モデルから0へ変化 （MWD⇒モデル時に不連続打消し分として使用） : simulink/Discontinuities/Rate Limiter Dynamic
  Subtract : Sum  Inputs=-+
  Switch1 : Switch  Threshold=1
  ∞ : Constant  Value=9999
  モデル使用時に レートを制限 : Switch  Threshold=1
  モデル使用時はモデル-MWD MWD使用時は0 : Switch  Threshold=1
  モデル使用時はモデル-MWDに追従 MWD使用時はレートでモデル-MWDから0に変化 （モデル⇒MWD時に不連続打消し分として使用） : simulink/Discontinuities/Rate Limiter Dynamic
  不連続 打消し分 : Switch  Threshold=1
  不連続分を戻すレート : Constant  Value=0.0001
  出力 : Outport  VectorParamsAs1DForOutWhenUnconnected=off
  wires:
  MWD/1 -> Subtract/2, Switch1/3
  モデル/1 -> Switch1/1, Subtract/1
  Constant/1 -> MWD使用時はMWD-モデル モデル使用時は0/1, モデル使用時はモデル-MWD MWD使用時は0/3
  Subtract/1 -> Gain2/1, MWD使用時はMWD-モデル モデル使用時は0/3
  MWD使用時はMWD-モデル モデル使用時は0/1 -> MWD使用時はMWD-モデルに追従 モデル使用時はレートでMWD-モデルから0へ変化 （MWD⇒モデル時に不連続打消し分として使用）/2
  モデル使用時はモデル-MWD MWD使用時は0/1 -> モデル使用時はモデル-MWDに追従 MWD使用時はレートでモデル-MWDから0に変化 （モデル⇒MWD時に不連続打消し分として使用）/2
  モデル使用時はモデル-MWDに追従 MWD使用時はレートでモデル-MWDから0に変化 （モデル⇒MWD時に不連続打消し分として使用）/1 -> 不連続 打消し分/3
  MWD使用時はMWD-モデルに追従 モデル使用時はレートでMWD-モデルから0へ変化 （MWD⇒モデル時に不連続打消し分として使用）/1 -> 不連続 打消し分/1
  Add/1 -> 出力/1
  不連続分を戻すレート/1 -> モデル使用時に レートを制限/1, MWD使用時に レートを制限/3
  ∞/1 -> モデル使用時に レートを制限/3, MWD使用時に レートを制限/1
  モデル使用時に レートを制限/1 -> MWD使用時はMWD-モデルに追従 モデル使用時はレートでMWD-モデルから0へ変化 （MWD⇒モデル時に不連続打消し分として使用）/1, Gain/1
  MWD使用時に レートを制限/1 -> モデル使用時はモデル-MWDに追従 MWD使用時はレートでモデル-MWDから0に変化 （モデル⇒MWD時に不連続打消し分として使用）/1, Gain1/1
  Gain/1 -> MWD使用時はMWD-モデルに追従 モデル使用時はレートでMWD-モデルから0へ変化 （MWD⇒モデル時に不連続打消し分として使用）/3
  Gain1/1 -> モデル使用時はモデル-MWDに追従 MWD使用時はレートでモデル-MWDから0に変化 （モデル⇒MWD時に不連続打消し分として使用）/3
  Gain2/1 -> モデル使用時はモデル-MWD MWD使用時は0/1
  Switch1/1 -> Add/1
  不連続 打消し分/1 -> Add/2
  運転モード/1 -> Switch1/2, MWD使用時はMWD-モデル モデル使用時は0/2, モデル使用時はモデル-MWD MWD使用時は0/2, モデル使用時に レートを制限/2, MWD使用時に レートを制限/2, 不連続 打消し分/2

== system AGC30_PVcut_2021/汽力プラント/Oil2/追従回路 ==
  In : Inport
  Subtract2 : Sum  Inputs=+-
  追従回路積分 : Integrator  InitialCondition=MW0_ST(2)/PTH0_ST(2)+PLM_ST(2)  LimitOutput=on  UpperSaturationLimit=U_LL_ST(2)  LowerSaturationLimit=L_LL_ST(2)
  追従変化率 : Saturate  UpperLimit=R_LL_ST(2)/60  LowerLimit=-R_LL_ST(2)/60
  追従時定数 : Gain  Gain=1/T_LL_ST(2)
  Out : Outport  VectorParamsAs1DForOutWhenUnconnected=off
  wires:
  Subtract2/1 -> 追従時定数/1
  追従時定数/1 -> 追従変化率/1
  追従変化率/1 -> 追従回路積分/1
  追従回路積分/1 -> Out/1, Subtract2/2
  In/1 -> Subtract2/1

== system AGC30_PVcut_2021/汽力プラント/Oil2/連続出力切替 ==
  モデル : Inport
  運転モード : Inport  Port=2
  MWD : Inport  Port=3
  Add : Sum
  Constant : Constant  Value=0
  Gain : Gain  Gain=-1
  Gain1 : Gain  Gain=-1
  Gain2 : Gain  Gain=-1
  MWD使用時に レートを制限 : Switch  Threshold=1
  MWD使用時はMWD-モデル モデル使用時は0 : Switch  Threshold=1
  MWD使用時はMWD-モデルに追従 モデル使用時はレートでMWD-モデルから0へ変化 （MWD⇒モデル時に不連続打消し分として使用） : simulink/Discontinuities/Rate Limiter Dynamic
  Subtract : Sum  Inputs=-+
  Switch1 : Switch  Threshold=1
  ∞ : Constant  Value=9999
  モデル使用時に レートを制限 : Switch  Threshold=1
  モデル使用時はモデル-MWD MWD使用時は0 : Switch  Threshold=1
  モデル使用時はモデル-MWDに追従 MWD使用時はレートでモデル-MWDから0に変化 （モデル⇒MWD時に不連続打消し分として使用） : simulink/Discontinuities/Rate Limiter Dynamic
  不連続 打消し分 : Switch  Threshold=1
  不連続分を戻すレート : Constant  Value=0.0001
  出力 : Outport  VectorParamsAs1DForOutWhenUnconnected=off
  wires:
  MWD/1 -> Subtract/2, Switch1/3
  モデル/1 -> Switch1/1, Subtract/1
  Constant/1 -> MWD使用時はMWD-モデル モデル使用時は0/1, モデル使用時はモデル-MWD MWD使用時は0/3
  Subtract/1 -> Gain2/1, MWD使用時はMWD-モデル モデル使用時は0/3
  MWD使用時はMWD-モデル モデル使用時は0/1 -> MWD使用時はMWD-モデルに追従 モデル使用時はレートでMWD-モデルから0へ変化 （MWD⇒モデル時に不連続打消し分として使用）/2
  モデル使用時はモデル-MWD MWD使用時は0/1 -> モデル使用時はモデル-MWDに追従 MWD使用時はレートでモデル-MWDから0に変化 （モデル⇒MWD時に不連続打消し分として使用）/2
  モデル使用時はモデル-MWDに追従 MWD使用時はレートでモデル-MWDから0に変化 （モデル⇒MWD時に不連続打消し分として使用）/1 -> 不連続 打消し分/3
  MWD使用時はMWD-モデルに追従 モデル使用時はレートでMWD-モデルから0へ変化 （MWD⇒モデル時に不連続打消し分として使用）/1 -> 不連続 打消し分/1
  Add/1 -> 出力/1
  不連続分を戻すレート/1 -> モデル使用時に レートを制限/1, MWD使用時に レートを制限/3
  ∞/1 -> モデル使用時に レートを制限/3, MWD使用時に レートを制限/1
  モデル使用時に レートを制限/1 -> MWD使用時はMWD-モデルに追従 モデル使用時はレートでMWD-モデルから0へ変化 （MWD⇒モデル時に不連続打消し分として使用）/1, Gain/1
  MWD使用時に レートを制限/1 -> モデル使用時はモデル-MWDに追従 MWD使用時はレートでモデル-MWDから0に変化 （モデル⇒MWD時に不連続打消し分として使用）/1, Gain1/1
  Gain/1 -> MWD使用時はMWD-モデルに追従 モデル使用時はレートでMWD-モデルから0へ変化 （MWD⇒モデル時に不連続打消し分として使用）/3
  Gain1/1 -> モデル使用時はモデル-MWDに追従 MWD使用時はレートでモデル-MWDから0に変化 （モデル⇒MWD時に不連続打消し分として使用）/3
  Gain2/1 -> モデル使用時はモデル-MWD MWD使用時は0/1
  Switch1/1 -> Add/1
  不連続 打消し分/1 -> Add/2
  運転モード/1 -> Switch1/2, MWD使用時はMWD-モデル モデル使用時は0/2, モデル使用時はモデル-MWD MWD使用時は0/2, モデル使用時に レートを制限/2, MWD使用時に レートを制限/2, 不連続 打消し分/2

== system AGC30_PVcut_2021/汽力プラント/Oil3/追従回路 ==
  In : Inport
  Subtract2 : Sum  Inputs=+-
  追従回路積分 : Integrator  InitialCondition=MW0_ST(3)/PTH0_ST(3)+PLM_ST(3)  UpperSaturationLimit=U_LL_ST(3)  LowerSaturationLimit=L_LL_ST(3)
  追従変化率 : Saturate  UpperLimit=R_LL_ST(3)/60  LowerLimit=-R_LL_ST(3)/60
  追従時定数 : Gain  Gain=1/T_LL_ST(3)
  Out : Outport  VectorParamsAs1DForOutWhenUnconnected=off
  wires:
  Subtract2/1 -> 追従時定数/1
  追従時定数/1 -> 追従変化率/1
  追従変化率/1 -> 追従回路積分/1
  追従回路積分/1 -> Out/1, Subtract2/2
  In/1 -> Subtract2/1

== system AGC30_PVcut_2021/汽力プラント/Oil3/連続出力切替 ==
  モデル : Inport
  運転モード : Inport  Port=2
  MWD : Inport  Port=3
  Add : Sum
  Constant : Constant  Value=0
  Gain : Gain  Gain=-1
  Gain1 : Gain  Gain=-1
  Gain2 : Gain  Gain=-1
  MWD使用時に レートを制限 : Switch  Threshold=1
  MWD使用時はMWD-モデル モデル使用時は0 : Switch  Threshold=1
  MWD使用時はMWD-モデルに追従 モデル使用時はレートでMWD-モデルから0へ変化 （MWD⇒モデル時に不連続打消し分として使用） : simulink/Discontinuities/Rate Limiter Dynamic
  Subtract : Sum  Inputs=-+
  Switch1 : Switch  Threshold=1
  ∞ : Constant  Value=9999
  モデル使用時に レートを制限 : Switch  Threshold=1
  モデル使用時はモデル-MWD MWD使用時は0 : Switch  Threshold=1
  モデル使用時はモデル-MWDに追従 MWD使用時はレートでモデル-MWDから0に変化 （モデル⇒MWD時に不連続打消し分として使用） : simulink/Discontinuities/Rate Limiter Dynamic
  不連続 打消し分 : Switch  Threshold=1
  不連続分を戻すレート : Constant  Value=0.0001
  出力 : Outport  VectorParamsAs1DForOutWhenUnconnected=off
  wires:
  MWD/1 -> Subtract/2, Switch1/3
  モデル/1 -> Switch1/1, Subtract/1
  Constant/1 -> MWD使用時はMWD-モデル モデル使用時は0/1, モデル使用時はモデル-MWD MWD使用時は0/3
  Subtract/1 -> Gain2/1, MWD使用時はMWD-モデル モデル使用時は0/3
  MWD使用時はMWD-モデル モデル使用時は0/1 -> MWD使用時はMWD-モデルに追従 モデル使用時はレートでMWD-モデルから0へ変化 （MWD⇒モデル時に不連続打消し分として使用）/2
  モデル使用時はモデル-MWD MWD使用時は0/1 -> モデル使用時はモデル-MWDに追従 MWD使用時はレートでモデル-MWDから0に変化 （モデル⇒MWD時に不連続打消し分として使用）/2
  モデル使用時はモデル-MWDに追従 MWD使用時はレートでモデル-MWDから0に変化 （モデル⇒MWD時に不連続打消し分として使用）/1 -> 不連続 打消し分/3
  MWD使用時はMWD-モデルに追従 モデル使用時はレートでMWD-モデルから0へ変化 （MWD⇒モデル時に不連続打消し分として使用）/1 -> 不連続 打消し分/1
  Add/1 -> 出力/1
  不連続分を戻すレート/1 -> モデル使用時に レートを制限/1, MWD使用時に レートを制限/3
  ∞/1 -> モデル使用時に レートを制限/3, MWD使用時に レートを制限/1
  モデル使用時に レートを制限/1 -> MWD使用時はMWD-モデルに追従 モデル使用時はレートでMWD-モデルから0へ変化 （MWD⇒モデル時に不連続打消し分として使用）/1, Gain/1
  MWD使用時に レートを制限/1 -> モデル使用時はモデル-MWDに追従 MWD使用時はレートでモデル-MWDから0に変化 （モデル⇒MWD時に不連続打消し分として使用）/1, Gain1/1
  Gain/1 -> MWD使用時はMWD-モデルに追従 モデル使用時はレートでMWD-モデルから0へ変化 （MWD⇒モデル時に不連続打消し分として使用）/3
  Gain1/1 -> モデル使用時はモデル-MWDに追従 MWD使用時はレートでモデル-MWDから0に変化 （モデル⇒MWD時に不連続打消し分として使用）/3
  Gain2/1 -> モデル使用時はモデル-MWD MWD使用時は0/1
  Switch1/1 -> Add/1
  不連続 打消し分/1 -> Add/2
  運転モード/1 -> Switch1/2, MWD使用時はMWD-モデル モデル使用時は0/2, モデル使用時はモデル-MWD MWD使用時は0/2, モデル使用時に レートを制限/2, MWD使用時に レートを制限/2, 不連続 打消し分/2

== system AGC30_PVcut_2021/汽力プラント/Oil4/追従回路 ==
  In : Inport
  Subtract2 : Sum  Inputs=+-
  追従回路積分1 : Integrator  InitialCondition=MW0_ST(4)/PTH0_ST(4)+PLM_ST(4)  LimitOutput=on  UpperSaturationLimit=U_LL_ST(4)  LowerSaturationLimit=L_LL_ST(4)
  追従変化率 : Saturate  UpperLimit=R_LL_ST(4)/60  LowerLimit=-R_LL_ST(4)/60
  追従時定数 : Gain  Gain=1/T_LL_ST(4)
  Out : Outport  VectorParamsAs1DForOutWhenUnconnected=off
  wires:
  Subtract2/1 -> 追従時定数/1
  追従時定数/1 -> 追従変化率/1
  追従変化率/1 -> 追従回路積分1/1
  追従回路積分1/1 -> Out/1, Subtract2/2
  In/1 -> Subtract2/1

== system AGC30_PVcut_2021/汽力プラント/Oil4/連続出力切替 ==
  モデル : Inport
  運転モード : Inport  Port=2
  MWD : Inport  Port=3
  Add : Sum
  Constant : Constant  Value=0
  Gain : Gain  Gain=-1
  Gain1 : Gain  Gain=-1
  Gain2 : Gain  Gain=-1
  MWD使用時に レートを制限 : Switch  Threshold=1
  MWD使用時はMWD-モデル モデル使用時は0 : Switch  Threshold=1
  MWD使用時はMWD-モデルに追従 モデル使用時はレートでMWD-モデルから0へ変化 （MWD⇒モデル時に不連続打消し分として使用） : simulink/Discontinuities/Rate Limiter Dynamic
  Subtract : Sum  Inputs=-+
  Switch1 : Switch  Threshold=1
  ∞ : Constant  Value=9999
  モデル使用時に レートを制限 : Switch  Threshold=1
  モデル使用時はモデル-MWD MWD使用時は0 : Switch  Threshold=1
  モデル使用時はモデル-MWDに追従 MWD使用時はレートでモデル-MWDから0に変化 （モデル⇒MWD時に不連続打消し分として使用） : simulink/Discontinuities/Rate Limiter Dynamic
  不連続 打消し分 : Switch  Threshold=1
  不連続分を戻すレート : Constant  Value=0.0001
  出力 : Outport  VectorParamsAs1DForOutWhenUnconnected=off
  wires:
  MWD/1 -> Subtract/2, Switch1/3
  モデル/1 -> Switch1/1, Subtract/1
  Constant/1 -> MWD使用時はMWD-モデル モデル使用時は0/1, モデル使用時はモデル-MWD MWD使用時は0/3
  Subtract/1 -> Gain2/1, MWD使用時はMWD-モデル モデル使用時は0/3
  MWD使用時はMWD-モデル モデル使用時は0/1 -> MWD使用時はMWD-モデルに追従 モデル使用時はレートでMWD-モデルから0へ変化 （MWD⇒モデル時に不連続打消し分として使用）/2
  モデル使用時はモデル-MWD MWD使用時は0/1 -> モデル使用時はモデル-MWDに追従 MWD使用時はレートでモデル-MWDから0に変化 （モデル⇒MWD時に不連続打消し分として使用）/2
  モデル使用時はモデル-MWDに追従 MWD使用時はレートでモデル-MWDから0に変化 （モデル⇒MWD時に不連続打消し分として使用）/1 -> 不連続 打消し分/3
  MWD使用時はMWD-モデルに追従 モデル使用時はレートでMWD-モデルから0へ変化 （MWD⇒モデル時に不連続打消し分として使用）/1 -> 不連続 打消し分/1
  Add/1 -> 出力/1
  不連続分を戻すレート/1 -> モデル使用時に レートを制限/1, MWD使用時に レートを制限/3
  ∞/1 -> モデル使用時に レートを制限/3, MWD使用時に レートを制限/1
  モデル使用時に レートを制限/1 -> MWD使用時はMWD-モデルに追従 モデル使用時はレートでMWD-モデルから0へ変化 （MWD⇒モデル時に不連続打消し分として使用）/1, Gain/1
  MWD使用時に レートを制限/1 -> モデル使用時はモデル-MWDに追従 MWD使用時はレートでモデル-MWDから0に変化 （モデル⇒MWD時に不連続打消し分として使用）/1, Gain1/1
  Gain/1 -> MWD使用時はMWD-モデルに追従 モデル使用時はレートでMWD-モデルから0へ変化 （MWD⇒モデル時に不連続打消し分として使用）/3
  Gain1/1 -> モデル使用時はモデル-MWDに追従 MWD使用時はレートでモデル-MWDから0に変化 （モデル⇒MWD時に不連続打消し分として使用）/3
  Gain2/1 -> モデル使用時はモデル-MWD MWD使用時は0/1
  Switch1/1 -> Add/1
  不連続 打消し分/1 -> Add/2
  運転モード/1 -> Switch1/2, MWD使用時はMWD-モデル モデル使用時は0/2, モデル使用時はモデル-MWD MWD使用時は0/2, モデル使用時に レートを制限/2, MWD使用時に レートを制限/2, 不連続 打消し分/2

== system AGC30_PVcut_2021/GTCCプラント/GTCC1/ガスタービン/出力特性 ==
  大気温度 : Inport
  圧縮機出口温度 : Inport  Port=2
  ガスタービン入口温度 : Inport  Port=3
  排ガス温度 : Inport  Port=4
  空気流量 : Inport  Port=5
  Add1 : Sum  Inputs=+--+
  Product2 : Product  Inputs=3  RndMeth=Zero
  ガスタービン出力係数 : Constant  Value=KGT_CC(1)
  ガスタービン出力 : Outport  VectorParamsAs1DForOutWhenUnconnected=off
  wires:
  Add1/1 -> Product2/1
  ガスタービン入口温度/1 -> Add1/1
  排ガス温度/1 -> Add1/2
  圧縮機出口温度/1 -> Add1/3
  大気温度/1 -> Add1/4
  空気流量/1 -> Product2/2
  ガスタービン出力係数/1 -> Product2/3
  Product2/1 -> ガスタービン出力/1

== system AGC30_PVcut_2021/GTCCプラント/GTCC1/ガスタービン/温度特性 ==
  燃料流量 : Inport
  空気流量 : Inport  Port=2
  ガスタービン入口温度算出部 : Subsystem
  圧縮機出口温度算出部 : Subsystem
  排ガス温度算出部 : Subsystem
  大気温度 : Outport  VectorParamsAs1DForOutWhenUnconnected=off
  圧縮機出口温度 : Outport  Port=2  VectorParamsAs1DForOutWhenUnconnected=off
  ガスタービン入口温度 : Outport  Port=3  VectorParamsAs1DForOutWhenUnconnected=off
  排ガス温度 : Outport  Port=4  VectorParamsAs1DForOutWhenUnconnected=off
  wires:
  圧縮機出口温度算出部/1(圧縮機出口温度) -> ガスタービン入口温度算出部/3(圧縮機入口温度), 圧縮機出口温度/1
  空気流量/1 -> ガスタービン入口温度算出部/2(空気流量), 圧縮機出口温度算出部/1(空気流量), 排ガス温度算出部/2(空気流量)
  ガスタービン入口温度算出部/1(ガスタービン入口温度) -> ガスタービン入口温度/1, 排ガス温度算出部/1(ガスタービン入口温度)
  排ガス温度算出部/1(排ガス温度) -> 排ガス温度/1
  燃料流量/1 -> ガスタービン入口温度算出部/1(燃料流量)
  圧縮機出口温度算出部/2(大気温度) -> 大気温度/1

== system AGC30_PVcut_2021/GTCCプラント/GTCC1/ガスタービン/空気流量 ==
  IGV開度 : Inport
  周波数偏差 : Inport  Port=2
  Product : Product  Inputs=3
  定格周波数[pu] : Constant
  空気密度比 : Constant  Value=TIR_CC(1)/TI_CC(1)
  系統周波数[pu] : Sum
  空気流量 : Outport  VectorParamsAs1DForOutWhenUnconnected=off
  wires:
  周波数偏差/1 -> 系統周波数[pu]/1
  定格周波数[pu]/1 -> 系統周波数[pu]/2
  空気密度比/1 -> Product/3
  系統周波数[pu]/1 -> Product/2
  IGV開度/1 -> Product/1
  Product/1 -> 空気流量/1

== system AGC30_PVcut_2021/可変速揚水発電機/可変速揚水/揚水運転/励磁装置および発電電動機 ==
  In1 : Inport
  Out1 : Outport  VectorParamsAs1DForOutWhenUnconnected=off
  wires:
  In1/1 -> Out1/1

== system AGC30_PVcut_2021/可変速揚水発電機/可変速揚水/発電運転/励磁装置および発電電動機 ==
  In1 : Inport
  Out1 : Outport  VectorParamsAs1DForOutWhenUnconnected=off
  wires:
  In1/1 -> Out1/1

== system AGC30_PVcut_2021/GTCCプラント/GTCC1/ガスタービン/温度特性/ガスタービン入口温度算出部 ==
  燃料流量 : Inport
  空気流量 : Inport  Port=2
  圧縮機入口温度 : Inport  Port=3
  Add : Sum  Inputs=+-
  Add1 : Sum
  Divide1 : Product  Inputs=*/
  Product2 : Product
  定格出力時ガスタービン入口温度 : Constant  Value=TFR_CC(1)
  定格出力時圧縮機出口温度 : Constant  Value=TDR_CC(1)
  ガスタービン入口温度 : Outport  VectorParamsAs1DForOutWhenUnconnected=off
  wires:
  Divide1/1 -> Product2/1
  Add/1 -> Product2/2
  燃料流量/1 -> Divide1/1
  Product2/1 -> Add1/1
  圧縮機入口温度/1 -> Add1/2
  定格出力時圧縮機出口温度/1 -> Add/2
  定格出力時ガスタービン入口温度/1 -> Add/1
  空気流量/1 -> Divide1/2
  Add1/1 -> ガスタービン入口温度/1

== system AGC30_PVcut_2021/GTCCプラント/GTCC1/ガスタービン/温度特性/圧縮機出口温度算出部 ==
  空気流量 : Inport
  Add : Sum  Inputs=+-
  Add1 : Sum
  Constant1 : Constant  Value=1.0
  Constant2 : Constant  Value=1.0
  Divide1 : Product  Inputs=*/
  Product2 : Product  RndMeth=Zero
  Product3 : Product  RndMeth=Zero
  pow : Math  Operator=pow  SignedPower=on  OutputSignalType=real  SaturateOnIntegerOverflow=on
  圧縮機入口温度 : Constant  Value=TI_CC(1)
  圧縮機効率 : Constant  Value=HC_CC(1)
  圧縮機圧力比 : Constant  Value=PRC_CC(1)
  比熱比 : Constant  Value=(RC_CC(1)-1)/RC_CC(1)
  圧縮機出口温度 : Outport  VectorParamsAs1DForOutWhenUnconnected=off
  大気温度 : Outport  Port=2  VectorParamsAs1DForOutWhenUnconnected=off
  wires:
  Constant2/1 -> Add1/2
  圧縮機圧力比/1 -> Product2/1
  pow/1 -> Add/1
  空気流量/1 -> Product2/2
  比熱比/1 -> pow/2
  Product2/1 -> pow/1
  Add/1 -> Divide1/1
  圧縮機効率/1 -> Divide1/2
  Constant1/1 -> Add/2
  Divide1/1 -> Add1/1
  Product3/1 -> 圧縮機出口温度/1
  Add1/1 -> Product3/1
  圧縮機入口温度/1 -> 大気温度/1, Product3/2

== system AGC30_PVcut_2021/GTCCプラント/GTCC1/ガスタービン/温度特性/排ガス温度算出部 ==
  ガスタービン入口温度 : Inport
  空気流量 : Inport  Port=2
  Add : Sum  Inputs=+-
  Add1 : Sum  Inputs=+-
  Constant1 : Constant  Value=1.0
  Divide1 : Product  Inputs=*/
  Product1 : Product  RndMeth=Zero
  Product2 : Product  RndMeth=Zero
  Product3 : Product  RndMeth=Zero
  pow : Math  Operator=pow  SignedPower=on  OutputSignalType=real  SaturateOnIntegerOverflow=on
  ガスタービン効率 : Constant  Value=HT_CC(1)
  ガスタービン圧力比 : Constant  Value=PRT_CC(1)
  比熱比 : Constant  Value=(RT_CC(1)-1)/RT_CC(1)
  排ガス温度 : Outport  VectorParamsAs1DForOutWhenUnconnected=off
  wires:
  ガスタービン効率/1 -> Product2/2
  Product2/1 -> Add1/2
  Add/1 -> Product2/1
  Constant1/1 -> Divide1/1, Add1/1, Add/1
  Divide1/1 -> Add/2
  Add1/1 -> Product3/2
  ガスタービン入口温度/1 -> Product3/1
  Product3/1 -> 排ガス温度/1
  ガスタービン圧力比/1 -> Product1/1
  比熱比/1 -> pow/2
  Product1/1 -> pow/1
  空気流量/1 -> Product1/2
  pow/1 -> Divide1/2

== matlab function AGC30_PVcut_2021/LFCモデル/自エリア TBC方式/Embedded MATLAB Function ==
  data: u input; y output; XAR_A input
function y = fcn(u,XAR_A)
%#eml
if (u > XAR_A) || (u < -XAR_A)
    y = u;
else
    y = 0.0;
end

== matlab function AGC30_PVcut_2021/LFCモデル/他エリア FFC方式/Embedded MATLAB Function5 ==
  data: u input; y output; XAR_B input
function y = fcn(u,XAR_B)
%#eml
if (u > XAR_B) || (u < -XAR_B)
    y = u;
else
    y = 0.0;
end

== matlab function AGC30_PVcut_2021/LFCモデル/自エリアFFC方式/Embedded MATLAB Function ==
  data: u input; y output; XAR_A input
function y = fcn(u,XAR_A)
%#eml
if (u > XAR_A) || (u < -XAR_A)
    y = u;
else
    y = 0.0;
end

== matlab function AGC30_PVcut_2021/LFCモデル/自エリアFFC方式/Embedded MATLAB Function1 ==
  data: u input; y output; XF_A input
function y = fcn(u,XF_A)
%#eml
if (u > XF_A) || (u < -XF_A)
    y = u;
else
    y = 0.0;
end

== matlab function AGC30_PVcut_2021/LFCモデル/他エリア TBC方式/Embedded MATLAB Function3 ==
  data: u input; y output; XAR_B input
function y = fcn(u,XAR_B)
%#eml
if (u > XAR_B) || (u < -XAR_B)
    y = u;
else
    y = 0.0;
end

== matlab function AGC30_PVcut_2021/LFCモデル/他エリア FFC方式/Embedded MATLAB Function4 ==
  data: u input; y output; XF_B input
function y = fcn(u,XF_B)
%#eml
if (u > XF_B) || (u < -XF_B)
    y = u;
else
    y = 0.0;
end
